simulink model "example_smart_braking"  (R2019b)
settings: Solver=VariableStepAuto  StartTime=0.0  StopTime=10.0  RelTol=1e-3
PreLoadFcn:
  | m=2000;
  | b=500;
libraries: simulink x2
settings Model: Creator=obas  LastModifiedBy=GM-ROBOT
settings DataIOCC: ReturnWorkspaceOutputs=off
settings DebuggingCC: ArithmeticOperatorsInVariantConditions=warning
settings SFSimCC: CustomCodeUndefinedFunction=UseInterfaceOnly

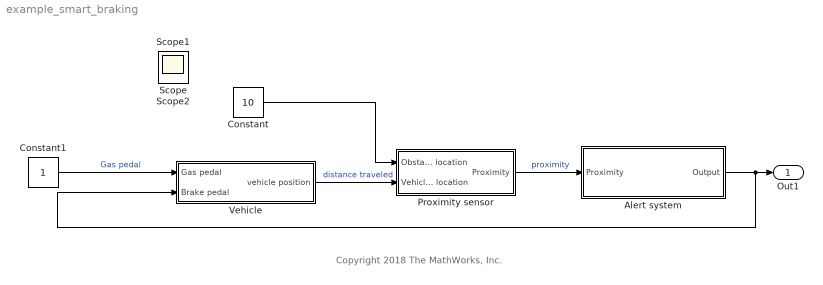
== system example_smart_braking ==
  note: Copyright 2018 The MathWorks, Inc.
  Alert system : Subsystem
  Constant : Constant  Value=10
  Constant1 : Constant
  Proximity sensor : Subsystem
  Vehicle : Subsystem
  Out1 : Outport  VectorParamsAs1DForOutWhenUnconnected=off
  Scope : Scope
  Scope1 : Scope
  Scope2 : Scope
  wires:
  Constant/1 -> Proximity sensor/1(Obstacle location)
  Vehicle/1(vehicle position) -> Proximity sensor/2(Vehicle location)  "distance traveled"
  Alert system/1(Output) -> Vehicle/2(Brake pedal), Out1/1
  Proximity sensor/1(Proximity) -> Alert system/1(Proximity)  "proximity"
  Constant1/1 -> Vehicle/1(Gas pedal)  "Gas pedal"

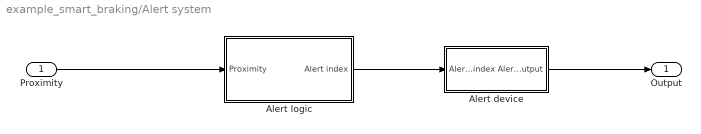
== system example_smart_braking/Alert system ==
  Proximity : Inport
  Alert device : Subsystem
  Alert logic : Subsystem
  Output : Outport  VectorParamsAs1DForOutWhenUnconnected=off
  wires:
  Proximity/1 -> Alert logic/1(Proximity)
  Alert logic/1(Alert index) -> Alert device/1(Alert index)
  Alert device/1(Alert output) -> Output/1

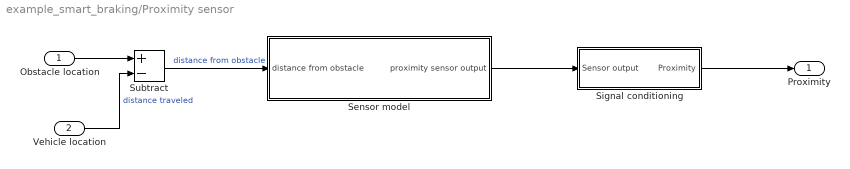
== system example_smart_braking/Proximity sensor ==
  Obstacle location : Inport
  Vehicle location : Inport  Port=2
  Sensor model : Subsystem
  Signal conditioning : Subsystem
  Subtract : Sum  Inputs=+-
  Proximity : Outport  VectorParamsAs1DForOutWhenUnconnected=off
  wires:
  Vehicle location/1 -> Subtract/2  "distance traveled"
  Obstacle location/1 -> Subtract/1
  Subtract/1 -> Sensor model/1(distance from obstacle)  "distance from obstacle"
  Signal conditioning/1(Proximity) -> Proximity/1
  Sensor model/1(proximity sensor output) -> Signal conditioning/1(Sensor output)

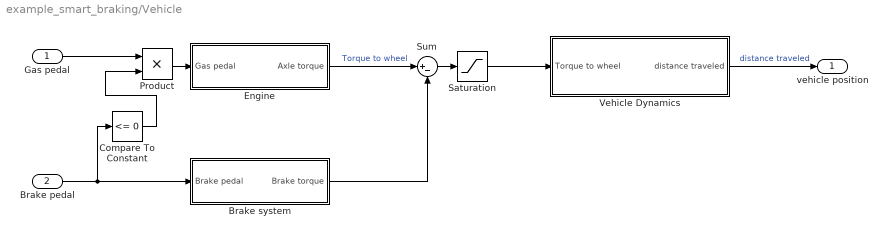
== system example_smart_braking/Vehicle ==
  Gas pedal : Inport
  Brake pedal : Inport  Port=2
  Brake system : Subsystem
  Compare To Constant : simulink/Logic and Bit Operations/Compare To Constant  relop=<=  const=0  OutDataTypeStr=boolean
  Engine : Subsystem
  Product : Product
  Saturation : Saturate  UpperLimit=inf  LowerLimit=0
  Sum : Sum  Inputs=|+-
  Vehicle Dynamics : Subsystem
  vehicle position : Outport  VectorParamsAs1DForOutWhenUnconnected=off
  wires:
  Vehicle Dynamics/1(distance traveled) -> vehicle position/1  "distance traveled"
  Brake pedal/1 -> Compare To Constant/1, Brake system/1(Brake pedal)
  Engine/1(Axle torque) -> Sum/1  "Torque to wheel"
  Sum/1 -> Saturation/1
  Brake system/1(Brake torque) -> Sum/2
  Saturation/1 -> Vehicle Dynamics/1(Torque to wheel)
  Product/1 -> Engine/1(Gas pedal)
  Gas pedal/1 -> Product/1
  Compare To Constant/1 -> Product/2

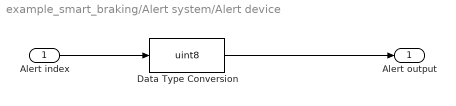
== system example_smart_braking/Alert system/Alert device ==
  Alert index : Inport
  Data Type Conversion : DataTypeConversion  OutDataTypeStr=uint8
  Alert output : Outport  VectorParamsAs1DForOutWhenUnconnected=off
  wires:
  Alert index/1 -> Data Type Conversion/1
  Data Type Conversion/1 -> Alert output/1

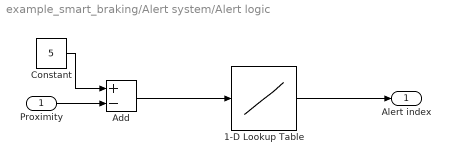
== system example_smart_braking/Alert system/Alert logic ==
  Proximity : Inport
  1-D Lookup Table : Lookup_n-D  NumberOfTableDimensions=1  BreakpointsForDimension1=0:0.4:2  BeginIndexSearchUsingPreviousIndexResult=on  Table=0:5  InterpMethod=Flat  InternalRulePriority=Speed  RndMeth=Simplest  InputSameDT=on
  Add : Sum  Inputs=+-
  Constant : Constant  Value=5
  Alert index : Outport  VectorParamsAs1DForOutWhenUnconnected=off
  wires:
  Constant/1 -> Add/1
  Proximity/1 -> Add/2
  Add/1 -> 1-D Lookup Table/1
  1-D Lookup Table/1 -> Alert index/1

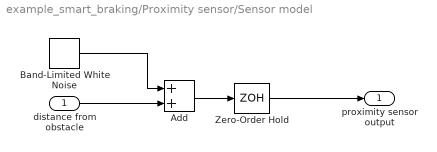
== system example_smart_braking/Proximity sensor/Sensor model ==
  distance from obstacle : Inport
  Add : Sum
  Band-Limited White Noise : simulink/Sources/Band-Limited White Noise  Cov=[0.001]  Ts=0.1  seed=[23341]
  Zero-Order Hold : ZeroOrderHold  SampleTime=0.1
  proximity sensor output : Outport  VectorParamsAs1DForOutWhenUnconnected=off
  wires:
  Band-Limited White Noise/1 -> Add/1
  Add/1 -> Zero-Order Hold/1
  distance from obstacle/1 -> Add/2
  Zero-Order Hold/1 -> proximity sensor output/1

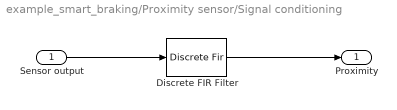
== system example_smart_braking/Proximity sensor/Signal conditioning ==
  Sensor output : Inport
  Discrete FIR Filter : DiscreteFir  Coefficients=ones(1,10)/10  InitialStates=10
  Proximity : Outport  VectorParamsAs1DForOutWhenUnconnected=off
  wires:
  Sensor output/1 -> Discrete FIR Filter/1
  Discrete FIR Filter/1 -> Proximity/1

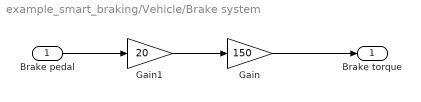
== system example_smart_braking/Vehicle/Brake system ==
  Brake pedal : Inport
  Gain : Gain  Gain=150
  Gain1 : Gain  Gain=20
  Brake torque : Outport  VectorParamsAs1DForOutWhenUnconnected=off
  wires:
  Gain/1 -> Brake torque/1
  Brake pedal/1 -> Gain1/1
  Gain1/1 -> Gain/1

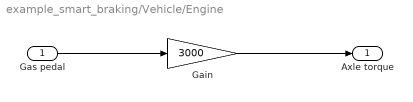
== system example_smart_braking/Vehicle/Engine ==
  Gas pedal : Inport
  Gain : Gain  Gain=3000
  Axle torque : Outport  VectorParamsAs1DForOutWhenUnconnected=off
  wires:
  Gas pedal/1 -> Gain/1
  Gain/1 -> Axle torque/1

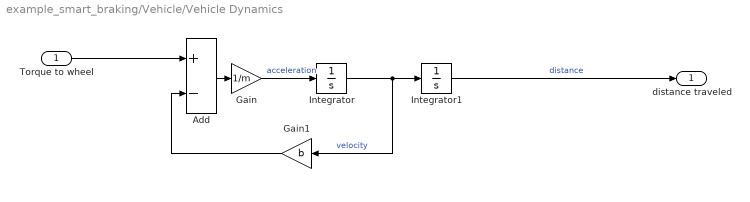
== system example_smart_braking/Vehicle/Vehicle Dynamics ==
  Torque to wheel : Inport
  Add : Sum  Inputs=+-
  Gain : Gain  Gain=1/m
  Gain1 : Gain  Gain=b
  Integrator : Integrator
  Integrator1 : Integrator
  distance traveled : Outport  VectorParamsAs1DForOutWhenUnconnected=off
  wires:
  Gain/1 -> Integrator/1  "acceleration"
  Integrator1/1 -> distance traveled/1  "distance"
  Gain1/1 -> Add/2
  Add/1 -> Gain/1
  Integrator/1 -> Gain1/1, Integrator1/1  "velocity"
  Torque to wheel/1 -> Add/1
